simulink library "kif2"  (R2022a)
settings: Solver=VariableStepAuto  StartTime=0.0  StopTime=10.0  RelTol=1e-3
undefined symbols (not defined in the file or in its folder): DiscIntNeverNeededParam
libraries: $bdroot x9, spsThreePhaseDynamicLoadLib x1, spsThreePhaseSeriesRLCLoadLib x1, spsGroundLib x1, spsControlledCurrentSourceLib x1, spsFourierLib x1, spsPLLLib x1, spsSeriesRLCBranchLib x1, spsVoltageMeasurementLib x1, spsThreePhasePISectionLineLib x1, spsThreePhaseVIMeasurementLib x1
settings Model: Creator=Felhasználó  LastModifiedBy=Felhasználó

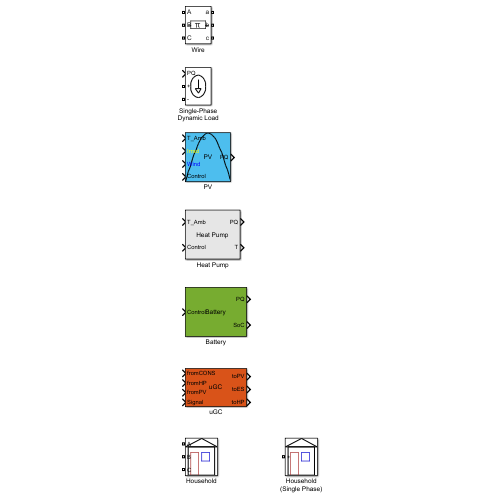
[thumbnail: Simulink's stored preview of the top-level diagram]
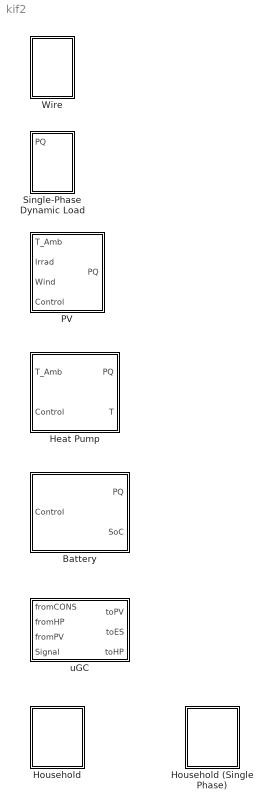
== system kif2 ==
  Battery : Subsystem  mask(Battery (Three Phase)){Cap=5000, SoCin=0.5, SoCmin=0.2, SoCmax=0.8, Pin=500, eta_in=0.95, Pout=-500, eta_out=0.95}
      mask prompts: Cap "Capacity (Wh)"; SoCin "Initial SoC (%)"; SoCmin "Min. SoC (%)"; SoCmax "Max. SoC (%)"; Pin "Max. charging power (W)"; eta_in "Charging efficiency (%)"; Pout "Max. discharging power (W)"; eta_out "Discharging efficiency (%)"
      mask help: This block models a battery.
      mask Display: disp('Battery');
  Heat Pump : Subsystem  mask(Heat Pump (Three Phase)){MFSystemSampleTime=0.05, tequiv=3, P_HP=3800, Tset=21, T_init=21, C=5940, H=192, ASHP=on, Mode=on, coeffs=[0.0012, -0.18, 8.6712], cosfi=0.9}
      mask prompts: MFSystemSampleTime "Simulink:blkprm_prompts:AllBlksSampleTime"; tequiv "Equivalent time (minutes)"; P_HP "Heat pump power (W)"; Tset "Set temperature (°C)"; T_init "Initial Temperature (°C)"; C "Building heat capacity (Wh/K)"; H "Building heat loss coefficient (W/K)"; ASHP "Air source heat pump"; Mode "Heating (/Cooling)"; coeffs "COP coefficients [a2 a1 a0]"; cosfi "Power factor (cosfi)"
      mask help: This block models an SG-Ready AHSP/WSHP/GSHP heat pump.
      mask TypeOptions MFSystemSampleTime: MATLAB Function/SystemSampleTime
      mask DialogControl MFSystemSampleTime Prompt: Sample time (-1 for inherited):
      mask Display: disp('Heat Pump');
  Household : Subsystem  mask(Household (Three Phase)){Ctag=CONSxx, Atag=Signal, Itag=Irradiation, Ttag=T_Amb, Wtag=Wind, HHtag=PQ_HHxx, HHtagv=local, PVtag=PQ_PVxx, PVtagv=local, EStag=PQ_ESxx, EStagv=local, HPtag=PQ_HPxx, HPtagv=local}
      mask prompts: Ctag "Consumption tag:"; Atag "Aggregator signal tag:"; Itag "Irradiation tag:"; Ttag "Temperature tag:"; Wtag "Wind tag:"; HHtag "Household:"; HHtagv "Simulink:blkprm_prompts:GotoTagVis"; PVtag "PV:"; PVtagv "Simulink:blkprm_prompts:GotoTagVis"; EStag "Battery:"; EStagv "Simulink:blkprm_prompts:GotoTagVis"; HPtag "Heat Pump:"; HPtagv "Simulink:blkprm_prompts:GotoTagVis"
      mask help: Represents a household, with PV, battery, heat pump and consumption.
      mask TypeOptions Ctag: Consumption/GotoTag
      mask TypeOptions Atag: Aggregator/GotoTag
      mask TypeOptions Itag: Irradiation/GotoTag
      mask TypeOptions Ttag: Temperature/GotoTag
      mask TypeOptions Wtag: Wind/GotoTag
      mask TypeOptions HHtag: PQ_HH/GotoTag
      mask TypeOptions HHtagv: PQ_HH/TagVisibility
      mask TypeOptions PVtag: PQ_PV/GotoTag
      mask TypeOptions PVtagv: PQ_PV/TagVisibility
      mask TypeOptions EStag: PQ_ES/GotoTag
      mask TypeOptions EStagv: PQ_ES/TagVisibility
      mask TypeOptions HPtag: PQ_HP/GotoTag
      mask TypeOptions HPtagv: PQ_HP/TagVisibility
      mask DialogControl InputTags Prompt: Inputs
      mask DialogControl WeatherTags Prompt: Weather
      mask DialogControl MeasurementTags Prompt: Measurement
      mask DialogControl HHtagv Prompt: Tag visibility:
      mask DialogControl PVtagv Prompt: Tag visibility:
      mask DialogControl EStagv Prompt: Tag visibility:
      mask DialogControl HPtagv Prompt: Tag visibility:
      mask Display:
      | plot([-5 -5 5 5 -5], [0 10 10 0 0]);
      | plot([-6 0 6 -6], [10 13 10 10]);
      | color('blue');
      | plot([0 3 3 0 0], [5 5 8 8 5]);
      | color('brown');
      | plot([-4 -1 -1 -4 -4], [0 0 8 8 0]);
  Household (Single Phase) : Subsystem  mask(Household (Single Phase)){Ctag=CONSxx, Atag=Signal, Itag=Irradiation, Ttag=T_Amb, Wtag=Wind, HHtag=PQ_HHxx, HHtagv=local, PVtag=PQ_PVxx, PVtagv=local, EStag=PQ_ESxx, EStagv=local, HPtag=PQ_HPxx, HPtagv=local}
      mask prompts: Ctag "Consumption tag:"; Atag "Aggregator signal tag:"; Itag "Irradiation tag:"; Ttag "Temperature tag:"; Wtag "Wind tag:"; HHtag "Household:"; HHtagv "Simulink:blkprm_prompts:GotoTagVis"; PVtag "PV:"; PVtagv "Simulink:blkprm_prompts:GotoTagVis"; EStag "Battery:"; EStagv "Simulink:blkprm_prompts:GotoTagVis"; HPtag "Heat Pump:"; HPtagv "Simulink:blkprm_prompts:GotoTagVis"
      mask help: Represents a Single Phase Household, with PV, battery, heat pump and consumption.
      mask TypeOptions Ctag: Consumption/GotoTag
      mask TypeOptions Atag: Aggregator/GotoTag
      mask TypeOptions Itag: Irradiation/GotoTag
      mask TypeOptions Ttag: Temperature/GotoTag
      mask TypeOptions Wtag: Wind/GotoTag
      mask TypeOptions HHtag: PQ_HH/GotoTag
      mask TypeOptions HHtagv: PQ_HH/TagVisibility
      mask TypeOptions PVtag: PQ_PV/GotoTag
      mask TypeOptions PVtagv: PQ_PV/TagVisibility
      mask TypeOptions EStag: PQ_ES/GotoTag
      mask TypeOptions EStagv: PQ_ES/TagVisibility
      mask TypeOptions HPtag: PQ_HP/GotoTag
      mask TypeOptions HPtagv: PQ_HP/TagVisibility
      mask DialogControl InputTags Prompt: Inputs
      mask DialogControl WeatherTags Prompt: Weather
      mask DialogControl MeasurementTags Prompt: Measurement
      mask DialogControl HHtagv Prompt: Tag visibility:
      mask DialogControl PVtagv Prompt: Tag visibility:
      mask DialogControl EStagv Prompt: Tag visibility:
      mask DialogControl HPtagv Prompt: Tag visibility:
      mask Display:
      | plot([-5 -5 5 5 -5], [0 10 10 0 0]);
      | plot([-6 0 6 -6], [10 13 10 10]);
      | color('blue');
      | plot([0 3 3 0 0], [5 5 8 8 5]);
      | color('brown');
      | plot([-4 -1 -1 -4 -4], [0 0 8 8 0]);
  PV : Subsystem  mask(PV (Three Phase)){P_STCm=2500, Ucoeff=[6.2 26.9], Kcoeff=[0.000005 0.00017 0.000149 -0.004702 -0.040465 -0.017237]}
      mask prompts: P_STCm "Peak Power (W)"; Ucoeff "Module temperature coefficients [u1 u0]"; Kcoeff "PV power dependence on irradiance and module temperature [k6 k5 k4 k3 k2 k1]"
      mask help: This block models a photovoltaic array.
      mask init:
      | U1 = Ucoeff(1);
      |     U0 = Ucoeff(2);
      |     k6 = Kcoeff(1);
      |     k5 = Kcoeff(2);
      |     k4 = Kcoeff(3);
      |     k3 = Kcoeff(4);
      |     k2 = Kcoeff(5);
      |     k1 = Kcoeff(6);
      mask Help: https://joint-research-centre.ec.europa.eu/photovoltaic-geographical-information-system-pvgis/getting-started-pvgis/pvgis-data-sources-calculation-methods_en
      mask Display:
      | disp('PV');
      | plot(-pi/2:0.1:pi/2, cos(-pi/2:0.1:pi/2));
  Single-Phase Dynamic Load : Subsystem  mask(Single-Phase Dynamic Load){Freq=50}
      mask prompts: Freq "Fundamental frequency (Hz):"
      mask help: This block models a PQ controlled single phase dynamic load.
      mask TypeOptions Freq: Fourier/Freq
      mask DialogControl ParameterGroupVar Prompt: PLL
      mask Display:
      | plot(-45,-45,45,45,[0,9,18,24,29,30,29,24,18,9,0,-9,-18,-24,-29,-30,-29,-24,-18,-9,0]*.9,[30,29,24,18,9,0,-9,-18,-24,-29,-30,-29,-24,-18,-9,0,9,18,24,29,30]*.9)
      | plot([0,0,10,0,-10,0]*1.1,[15,-5,-5,-15,-5,-5]*1.1)
  Wire : Subsystem  mask(Three-Phase Low Voltage Distribution Line){Length=0.03, Frequency=50, Resistances=[0.2968 0.4468], Inductances=[0.95359e-3  5.4671e-3], Capacitances=[12.458e-9 3.9055e-9], Vtag=V_Lxx, Vtagv=local, Itag=I_Lxx, Itagv=local}
      mask prompts: Length "Line length (km):"; Frequency "Frequency used for rlc specification (Hz):"; Resistances "Positive- and zero-sequence resistances (Ohms/km) [ r1  r0 ]:"; Inductances "Positive- and zero-sequence inductances (H/km) [ l1  l0 ]:"; Capacitances "Positive- and zero-sequence capacitances (F/km) [ c1 c0 ]:"; Vtag "V tag"; Vtagv "Visibility"; Itag "I tag"; Itagv "Visibility"
      mask help: This block models a low voltage distribution line with a Three-Phase PI Section Line, corresponding ports and V-I measurement.
      mask TypeOptions Length:
      | Three-Phase
      | PI Section Line/Length
      mask TypeOptions Frequency:
      | Three-Phase
      | PI Section Line/Frequency
      mask TypeOptions Resistances:
      | Three-Phase
      | PI Section Line/Resistances
      mask TypeOptions Inductances:
      | Three-Phase
      | PI Section Line/Inductances
      mask TypeOptions Capacitances:
      | Three-Phase
      | PI Section Line/Capacitances
      mask TypeOptions Vtag: Vmeas/GotoTag
      mask TypeOptions Vtagv: Vmeas/TagVisibility
      mask TypeOptions Itag: Imeas/GotoTag
      mask TypeOptions Itagv: Imeas/TagVisibility
      mask DialogControl Container3 Prompt: Measurements
      mask Display: block_icon('Three-Phase PI Section Line');
  uGC : Subsystem  mask(Microgrid Controller){}
      mask help: This block models a microgrid controller. It accepts aggregator signals, and controls PV, battery and heat pump.
      mask Display: disp('uGC');

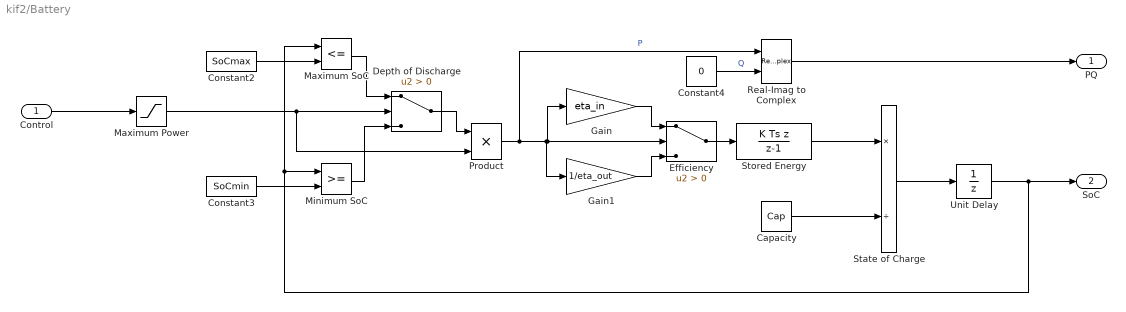
== system kif2/Battery ==
  Control : Inport
  Capacity : Constant  Value=Cap
  Constant2 : Constant  Value=SoCmax
  Constant3 : Constant  Value=SoCmin
  Constant4 : Constant  Value=0
  Depth of Discharge : Switch  Criteria=u2 > Threshold  SaturateOnIntegerOverflow=off  InputSameDT=off
  Efficiency : Switch  Criteria=u2 > Threshold  SaturateOnIntegerOverflow=off  InputSameDT=off
  Gain : Gain  Gain=eta_in
  Gain1 : Gain  Gain=1/eta_out
  Maximum Power : Saturate  UpperLimit=Pin  LowerLimit=Pout
  Maximum SoC : RelationalOperator  Operator=<=  OutDataTypeStr=boolean  RndMeth=Simplest  InputSameDT=off
  Minimum SoC : RelationalOperator  OutDataTypeStr=boolean  RndMeth=Simplest  InputSameDT=off
  Product : Product
  Real-Imag to Complex : RealImagToComplex
  State of Charge : Product  Inputs=*/
  Stored Energy : DiscreteIntegrator  IntegratorMethod=Integration: Backward Euler  InitialCondition=Cap*SoCin  SampleTime=1e-4  LimitOutput=on  UpperSaturationLimit=Cap  LowerSaturationLimit=0  ICPrevOutput=DiscIntNeverNeededParam  ICPrevScaledInput=DiscIntNeverNeededParam
  Unit Delay : UnitDelay  SampleTime=-1  HasFrameUpgradeWarning=on
  PQ : Outport
  SoC : Outport  Port=2
  wires:
  Control/1 -> Maximum Power/1
  Unit Delay/1 -> SoC/1, Maximum SoC/1, Minimum SoC/1
  Depth of Discharge/1 -> Product/1
  Product/1 -> Gain1/1, Gain/1, Efficiency/2, Real-Imag to Complex/1  "P"
  Constant4/1 -> Real-Imag to Complex/2  "Q"
  Maximum Power/1 -> Product/2, Depth of Discharge/2
  State of Charge/1 -> Unit Delay/1
  Constant2/1 -> Maximum SoC/2
  Stored Energy/1 -> State of Charge/1
  Maximum SoC/1 -> Depth of Discharge/1
  Capacity/1 -> State of Charge/2
  Minimum SoC/1 -> Depth of Discharge/3
  Constant3/1 -> Minimum SoC/2
  Real-Imag to Complex/1 -> PQ/1
  Efficiency/1 -> Stored Energy/1
  Gain/1 -> Efficiency/1
  Gain1/1 -> Efficiency/3

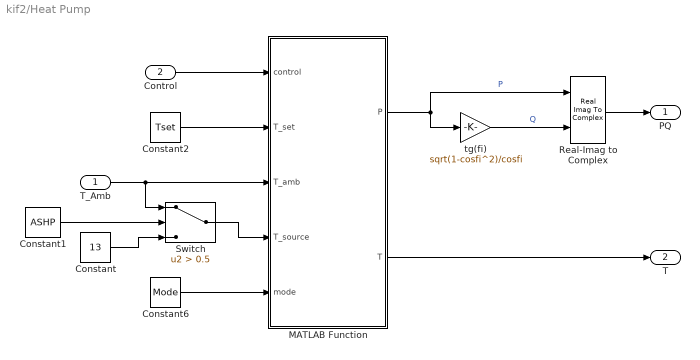
== system kif2/Heat Pump ==
  T_Amb : Inport
  Control : Inport  Port=2
  Constant : Constant  Value=13
  Constant1 : Constant  Value=ASHP
  Constant2 : Constant  Value=Tset
  Constant6 : Constant  Value=Mode
  MATLAB Function : MATLAB Function  TreatAsAtomicUnit=on  SystemSampleTime=MFSystemSampleTime
  Real-Imag to Complex : RealImagToComplex
  Switch : Switch  Criteria=u2 > Threshold  Threshold=0.5  SaturateOnIntegerOverflow=off  InputSameDT=off
  tg(fi) : Gain  Gain=sqrt(1-cosfi^2)/cosfi
  PQ : Outport
  T : Outport  Port=2
  wires:
  tg(fi)/1 -> Real-Imag to Complex/2  "Q"
  MATLAB Function/1(P) -> Real-Imag to Complex/1, tg(fi)/1  "P"
  T_Amb/1 -> Switch/1, MATLAB Function/3(T_amb)
  Constant2/1 -> MATLAB Function/2(T_set)
  Constant6/1 -> MATLAB Function/5(mode)
  Constant/1 -> Switch/3
  Switch/1 -> MATLAB Function/4(T_source)
  Constant1/1 -> Switch/2
  Control/1 -> MATLAB Function/1(control)
  MATLAB Function/2(T) -> T/1
  Real-Imag to Complex/1 -> PQ/1

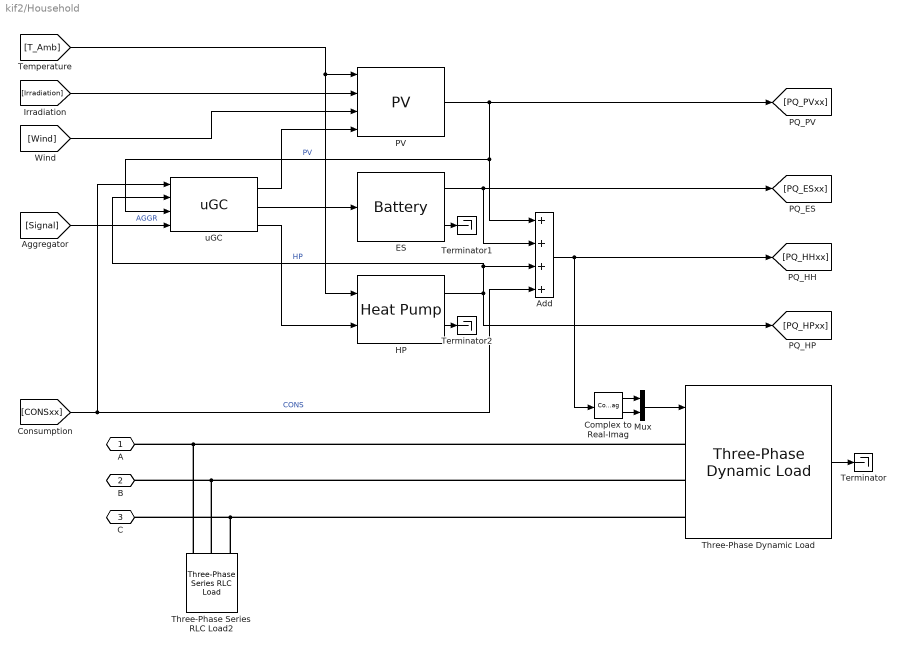
== system kif2/Household ==
  Add : Sum  Inputs=4
  Complex to Real-Imag : ComplexToRealImag
  ES : $bdroot/Battery  Cap=5000  SoCin=0.5  SoCmin=0.2  SoCmax=0.8  Pin=500  eta_in=0.95  Pout=-500  eta_out=0.95
  HP : $bdroot/Heat Pump  MFSystemSampleTime=0.05  tequiv=3  P_HP=3800  Tset=21  T_init=21  C=5940  H=192  ASHP=on  Mode=on  coeffs=[0.0012, -0.18, 8.6712]  cosfi=0.9
  Mux : Mux  Inputs=2
  PV : $bdroot/PV  P_STCm=2500  Ucoeff=[6.2 26.9]  Kcoeff=[0.000005 0.00017 0.000149 -0.004702 -0.040465 -0.017237]
  Terminator : Terminator
  Terminator1 : Terminator
  Terminator2 : Terminator
  Three-Phase Dynamic Load : spsThreePhaseDynamicLoadLib/Three-Phase Dynamic Load  NominalVoltage=[ 400 50 ]  ActiveReactivePowers=[0 0]  PositiveSequence=[0.994 -11.8]  ExternalControl=on  NpNq=[1.3 2]  TimeConstants="[0  0  0  0]"  MinimumVoltage=0.7  Tfilter=1e-4  LoadFlowParameters=[4,0,0,0,0]
      settings: SourceProductBaseCode=PS
  Three-Phase Series RLC Load2 : spsThreePhaseSeriesRLCLoadLib/Three-Phase Series RLC Load  LConnTagsString=A|B|C  Configuration=Y (grounded)  NominalVoltage=400  Vabc=[1e3 1e3 1e3]  Vabcp=[1e3 1e3 1e3]  NominalFrequency=50  UnbalancedPower=off  ActivePower=1  InductivePower=0  CapacitivePower=0  Pabc=[10e3 9e3 11e3]  QLabc=[100 90 110]  QCabc=[100 90 110]  Pabcp=[10e3 9e3 11e3]  QLabcp=[100 90 110]  QCabcp=[100 90 110]  Measurements=None  LoadType=constant Z
  uGC : $bdroot/uGC
  A : PMIOPort  Side=Left
  B : PMIOPort  Port=2  Side=Left
  C : PMIOPort  Port=3  Side=Left
  wires:
  Three-Phase Dynamic Load/1 -> Terminator/1
  Add/1 -> [PQ_HHxx], Complex to Real-Imag/1
  Complex to Real-Imag/1 -> Mux/1
  Complex to Real-Imag/2 -> Mux/2
  Mux/1 -> Three-Phase Dynamic Load/1
  PV/1 -> [PQ_PVxx], uGC/3, Add/1  "PV"
  [CONSxx] -> Add/4, uGC/1  "CONS"
  uGC/1 -> PV/4
  ES/1 -> [PQ_ESxx], Add/2
  HP/1 -> uGC/2, Add/3, [PQ_HPxx]  "HP"
  ES/2 -> Terminator1/1
  HP/2 -> Terminator2/1
  uGC/2 -> ES/1
  uGC/3 -> HP/2
  [Signal] -> uGC/4  "AGGR"
  [T_Amb] -> HP/1, PV/1
  [Irradiation] -> PV/2
  [Wind] -> PV/3
  connections:
  Three-Phase Dynamic Load/LConn1 -- A/RConn1 -- Three-Phase Series RLC Load2/LConn1
  Three-Phase Dynamic Load/LConn2 -- B/RConn1 -- Three-Phase Series RLC Load2/LConn2
  Three-Phase Dynamic Load/LConn3 -- C/RConn1 -- Three-Phase Series RLC Load2/LConn3

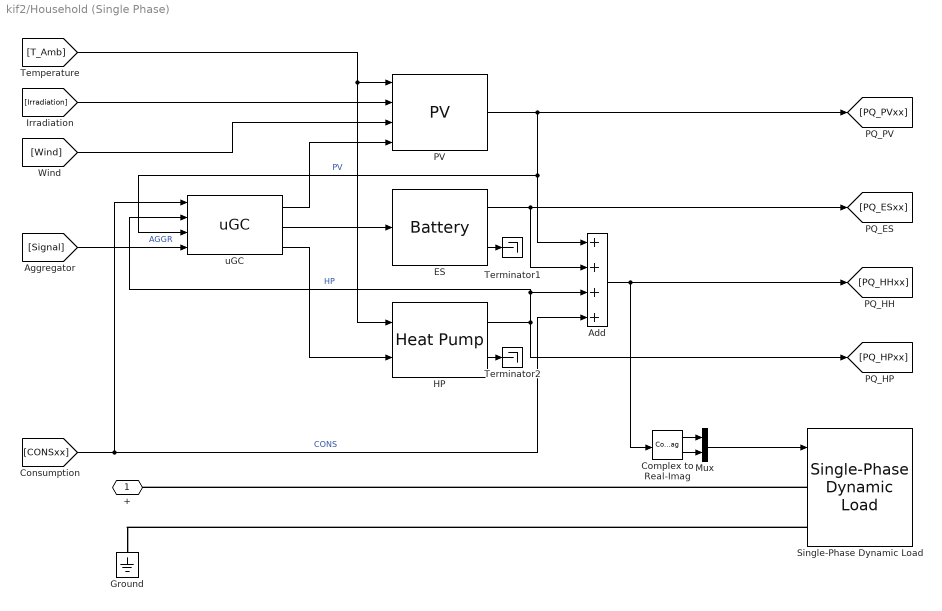
== system kif2/Household (Single Phase) ==
  Add : Sum  Inputs=4
  Complex to Real-Imag : ComplexToRealImag
  ES : $bdroot/Battery  Cap=5000  SoCin=0.5  SoCmin=0.2  SoCmax=0.8  Pin=500  eta_in=0.95  Pout=-500  eta_out=0.95
  Ground : spsGroundLib/Ground  LConnTagsString=a
  HP : $bdroot/Heat Pump  MFSystemSampleTime=0.05  tequiv=3  P_HP=3800  Tset=21  T_init=21  C=5940  H=192  ASHP=on  Mode=on  coeffs=[0.0012, -0.18, 8.6712]  cosfi=0.9
  Mux : Mux  Inputs=2
  PV : $bdroot/PV  P_STCm=2500  Ucoeff=[6.2 26.9]  Kcoeff=[0.000005 0.00017 0.000149 -0.004702 -0.040465 -0.017237]
  Single-Phase Dynamic Load : $bdroot/Single-Phase Dynamic Load  Freq=50
  Terminator1 : Terminator
  Terminator2 : Terminator
  uGC : $bdroot/uGC
  + : PMIOPort  Side=Left
  wires:
  [Wind] -> PV/3
  [Irradiation] -> PV/2
  [T_Amb] -> PV/1, HP/1
  [Signal] -> uGC/4  "AGGR"
  uGC/3 -> HP/2
  uGC/2 -> ES/1
  HP/2 -> Terminator2/1
  ES/2 -> Terminator1/1
  HP/1 -> [PQ_HPxx], Add/3, uGC/2  "HP"
  ES/1 -> Add/2, [PQ_ESxx]
  uGC/1 -> PV/4
  [CONSxx] -> Add/4, uGC/1  "CONS"
  PV/1 -> uGC/3, Add/1, [PQ_PVxx]  "PV"
  Mux/1 -> Single-Phase Dynamic Load/1
  Complex to Real-Imag/2 -> Mux/2
  Complex to Real-Imag/1 -> Mux/1
  Add/1 -> Complex to Real-Imag/1, [PQ_HHxx]
  connections:
  Single-Phase Dynamic Load/LConn1 -- +/RConn1
  Single-Phase Dynamic Load/LConn2 -- Ground/LConn1

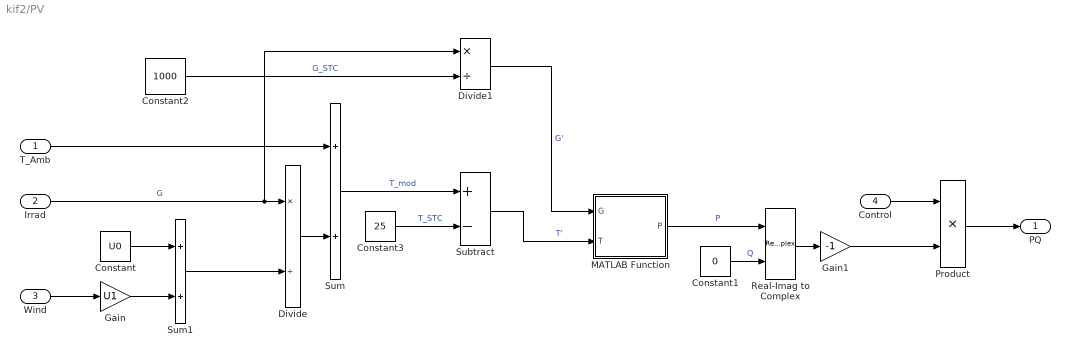
== system kif2/PV ==
  T_Amb : Inport
  Irrad : Inport  Port=2
  Wind : Inport  Port=3
  Control : Inport  Port=4
  Constant : Constant  Value=U0
  Constant1 : Constant  Value=0
  Constant2 : Constant  Value=1000
  Constant3 : Constant  Value=25
  Divide : Product  Inputs=*/
  Divide1 : Product  Inputs=*/
  Gain : Gain  Gain=U1
  Gain1 : Gain  Gain=-1
  MATLAB Function : MATLAB Function  TreatAsAtomicUnit=on
  Product : Product
  Real-Imag to Complex : RealImagToComplex
  Subtract : Sum  Inputs=+-
  Sum : Sum
  Sum1 : Sum
  PQ : Outport
  wires:
  Constant2/1 -> Divide1/2  "G_STC"
  Wind/1 -> Gain/1
  Irrad/1 -> Divide/1, Divide1/1  "G"
  T_Amb/1 -> Sum/1
  Constant3/1 -> Subtract/2  "T_STC"
  Sum/1 -> Subtract/1  "T_mod"
  Divide1/1 -> MATLAB Function/1(G)  "G'"
  Constant/1 -> Sum1/1
  Gain/1 -> Sum1/2
  Divide/1 -> Sum/2
  Sum1/1 -> Divide/2
  Subtract/1 -> MATLAB Function/2(T)  "T'"
  MATLAB Function/1(P) -> Real-Imag to Complex/1  "P"
  Constant1/1 -> Real-Imag to Complex/2  "Q"
  Control/1 -> Product/1
  Real-Imag to Complex/1 -> Gain1/1
  Product/1 -> PQ/1
  Gain1/1 -> Product/2

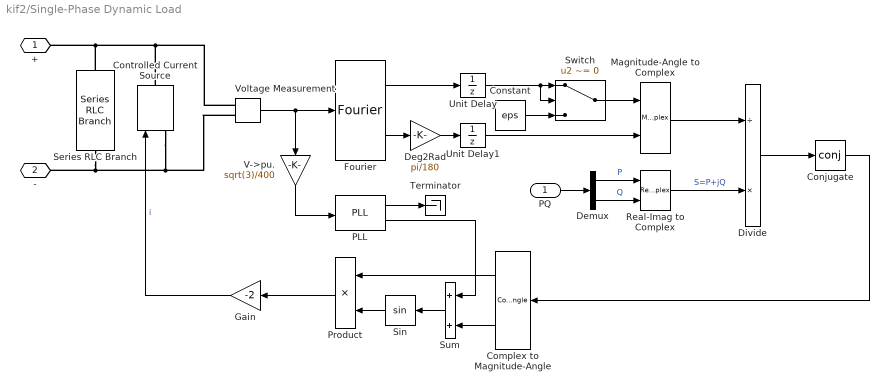
== system kif2/Single-Phase Dynamic Load ==
  PQ : Inport
  Complex to Magnitude-Angle : ComplexToMagnitudeAngle
  Conjugate : Math  Operator=conj  SignedPower=on  RndMeth=Zero
  Constant : Constant  Value=eps
  Controlled Current Source : spsControlledCurrentSourceLib/Controlled Current Source  Initialize=on  Source_Type=AC  Amplitude=0  Phase=0  Frequency=50  Measurements=None
  Deg2Rad : Gain  Gain=pi/180
  Demux : Demux  Outputs=2
  Divide : Product  Inputs=/*
  Fourier : spsFourierLib/Fourier  Freq=Freq  n=1  InInit=[400/sqrt(3), 0]  Ts=0
      settings: SourceProductBaseCode=PS
  Gain : Gain  Gain=-2
  Magnitude-Angle to Complex : MagnitudeAngleToComplex
  PLL : spsPLLLib/PLL  Fmin=45  Par_Init=[0, 50]  ParK=[180, 3200, 1]  TcD=1e-4  MaxRateChangeFreq=12  FilterCutOffFreq=25  Ts=0  AGC=on
      settings: SourceProductBaseCode=PS
  Product : Product
  Real-Imag to Complex : RealImagToComplex
  Series RLC Branch : spsSeriesRLCBranchLib/Series RLC Branch  LConnTagsString=__new0  RConnTagsString=__new0  BranchType=R  Resistance=1e6  Inductance=1e-3  SetiL0=off  InitialCurrent=0  Capacitance=1e-6  Setx0=off  InitialVoltage=0  Measurements=None
  Sin : Trigonometry
  Sum : Sum
  Switch : Switch  Criteria=u2 ~= 0  SaturateOnIntegerOverflow=off  InputSameDT=off
  Terminator : Terminator
  Unit Delay : UnitDelay  SampleTime=-1  HasFrameUpgradeWarning=on
  Unit Delay1 : UnitDelay  SampleTime=-1  HasFrameUpgradeWarning=on
  V->pu. : Gain  Gain=sqrt(3)/400
  Voltage Measurement : spsVoltageMeasurementLib/Voltage Measurement  PhasorSimulation=off  OutputType=Complex  PSBequivalent=0
  + : PMIOPort  Side=Left
  - : PMIOPort  Port=2  Side=Left
  wires:
  Divide/1 -> Conjugate/1
  Fourier/1 -> Unit Delay/1
  Complex to Magnitude-Angle/1 -> Product/1
  Magnitude-Angle to Complex/1 -> Divide/1
  Sum/1 -> Sin/1
  PQ/1 -> Demux/1
  Unit Delay1/1 -> Magnitude-Angle to Complex/2
  Voltage Measurement/1 -> V->pu./1, Fourier/1
  Constant/1 -> Switch/3
  PLL/1 -> Terminator/1
  Demux/1 -> Real-Imag to Complex/1  "P"
  Unit Delay/1 -> Switch/2, Switch/1
  Complex to Magnitude-Angle/2 -> Sum/2
  Sin/1 -> Product/2
  Product/1 -> Gain/1
  Real-Imag to Complex/1 -> Divide/2  "S=P+jQ"
  Fourier/2 -> Deg2Rad/1
  Conjugate/1 -> Complex to Magnitude-Angle/1
  Gain/1 -> Controlled Current Source/1  "i"
  Switch/1 -> Magnitude-Angle to Complex/1
  Demux/2 -> Real-Imag to Complex/2  "Q"
  PLL/2 -> Sum/1
  Deg2Rad/1 -> Unit Delay1/1
  V->pu./1 -> PLL/1
  connections:
  Voltage Measurement/LConn2 -- Controlled Current Source/LConn1 -- -/RConn1 -- Series RLC Branch/RConn1
  Voltage Measurement/LConn1 -- +/RConn1 -- Series RLC Branch/LConn1 -- Controlled Current Source/RConn1

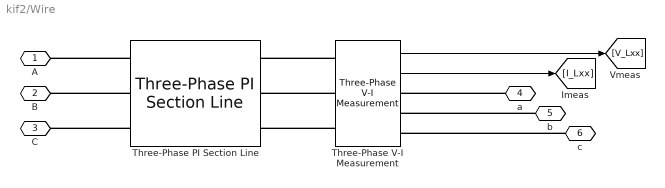
== system kif2/Wire ==
  Three-Phase PI Section Line : spsThreePhasePISectionLineLib/Three-Phase PI Section Line  LConnTagsString=a|b|c  RConnTagsString=A|B|C  Length=Length  Frequency=Frequency  Resistances=Resistances  Inductances=Inductances  Capacitances=Capacitances
  Three-Phase V-I Measurement : spsThreePhaseVIMeasurementLib/Three-Phase V-I Measurement  VoltageMeasurement=phase-to-ground  SetLabelV=off  LabelV=Vabc  Vpu=off  VpuLL=off  CurrentMeasurement=yes  SetLabelI=off  LabelI=Iabc  Ipu=off  Pbase=100e6  Vbase=500e3  OutputType=Complex  PhasorSimulation=off  PSBequivalent=0
  A : PMIOPort  Side=Left
  B : PMIOPort  Port=2  Side=Left
  C : PMIOPort  Port=3  Side=Left
  a : PMIOPort  Port=4  Side=Right
  b : PMIOPort  Port=5  Side=Right
  c : PMIOPort  Port=6  Side=Right
  wires:
  Three-Phase V-I Measurement/1 -> [V_Lxx]
  Three-Phase V-I Measurement/2 -> [I_Lxx]
  connections:
  c/RConn1 -- Three-Phase V-I Measurement/RConn3
  Three-Phase PI Section Line/LConn3 -- C/RConn1
  Three-Phase V-I Measurement/LConn3 -- Three-Phase PI Section Line/RConn3
  b/RConn1 -- Three-Phase V-I Measurement/RConn2
  Three-Phase V-I Measurement/LConn2 -- Three-Phase PI Section Line/RConn2
  a/RConn1 -- Three-Phase V-I Measurement/RConn1
  Three-Phase PI Section Line/LConn2 -- B/RConn1
  Three-Phase PI Section Line/LConn1 -- A/RConn1
  Three-Phase V-I Measurement/LConn1 -- Three-Phase PI Section Line/RConn1

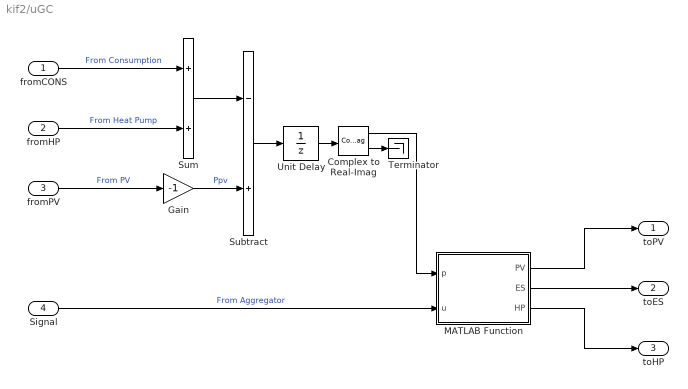
== system kif2/uGC ==
  fromCONS : Inport
  fromHP : Inport  Port=2
  fromPV : Inport  Port=3
  Signal : Inport  Port=4
  Complex to Real-Imag : ComplexToRealImag
  Gain : Gain  Gain=-1
  MATLAB Function : MATLAB Function  TreatAsAtomicUnit=on
  Subtract : Sum  Inputs=-+
  Sum : Sum
  Terminator : Terminator
  Unit Delay : UnitDelay  SampleTime=-1  HasFrameUpgradeWarning=on
  toPV : Outport
  toES : Outport  Port=2
  toHP : Outport  Port=3
  wires:
  Sum/1 -> Subtract/1
  Subtract/1 -> Unit Delay/1
  MATLAB Function/3(HP) -> toHP/1
  MATLAB Function/1(PV) -> toPV/1
  MATLAB Function/2(ES) -> toES/1
  fromCONS/1 -> Sum/1  "From Consumption"
  fromHP/1 -> Sum/2  "From Heat Pump"
  fromPV/1 -> Gain/1  "From PV"
  Signal/1 -> MATLAB Function/2(u)  "From Aggregator"
  Gain/1 -> Subtract/2  "Ppv"
  Unit Delay/1 -> Complex to Real-Imag/1
  Complex to Real-Imag/1 -> MATLAB Function/1(p)
  Complex to Real-Imag/2 -> Terminator/1

== matlab function kif2/PV/MATLAB Function ==
  data: G input; P output; T input; P_STCm parameter; k1 parameter; k2 parameter; k3 parameter; k4 parameter; k5 parameter; k6 parameter
function P = fcn(G,T, P_STCm, k1, k2, k3, k4, k5, k6)
    if G < eps
        P = 0;
    else
        P = G*(P_STCm + k1*log(G) + k2*log(G)^2 + k3*T + k4*T*log(G) + k5*T*log(G)^2 + k6*T^2);
    end
end

== matlab function kif2/Heat Pump/MATLAB Function ==
  data: P output; control input; T_set input; T_amb input; T_source input; mode input; T output; P_HP parameter; H parameter; C parameter; coeffs parameter; T_init parameter; tequiv parameter
% OFF = 1
% NORMAL = 2
% ON = 3
% SUPERHEAT_A = 4
% SUPERHEAT_B = 5

function [P, T] = fcn(control, T_set, T_amb, T_source, mode, P_HP, H, C, coeffs, T_init, tequiv)
    HYST = 0.5;
    HYST_adj = 1;
    min_run_time = 3;
    min_pause_time = 6;
    T_sink = 45;
    
    persistent pause_time;
    if isempty(pause_time)
        pause_time = 0;
    end
    persistent run_time;
    if isempty(run_time)
        run_time = 0;
    end
    persistent on;
    if isempty(on)
        on = false;
    end
    persistent prev_control;
    if isempty(prev_control)
        prev_control = 2;
    end
    
    persistent T_in;
    if isempty(T_in)
        T_in = T_init;
    end
    
    %initial values
    Q_HP = 0;
    %default hysteresis
    T_min = T_set - HYST;
    T_max = T_set + HYST;
    
    if (mode) %heating
        %adjust histeresis based on control
        if (control == 3 || control >= 4)
            T_min = T_set;
            T_max = T_set + HYST + HYST_adj;
        end
        %switch on/off
        if (~on && ...
                pause_time >= min_pause_time && ...
                control ~= 1 && ...
                (T_in < T_min || (control >= 4 && prev_control < 4)))
            on = true;
            run_time = 0;
        elseif (on && ...
                run_time >= min_run_time && ...
                (T_in > T_max || control == 1))
            on = false;
            pause_time = 0;
        end
        %determine P and Q
        if (on)
            COP = polyval(coeffs, T_sink - T_source);
            Q_HP = P_HP * COP;
            P = P_HP;
            run_time = run_time + tequiv;
        else
            P = 0;
            pause_time = pause_time + tequiv;
        end
    else %cooling
        %adjust histeresis based on control
        if (control == 3 || control >= 4)
            T_min = T_set - HYST - HYST_adj;
            T_max = T_set;
        end
        %switch on/off
        if (~on && ...
                pause_time >= min_pause_time && ...
                control ~= 1 && ...
                (T_in > T_max || (control >= 4 && prev_control < 4)))
            on = true;
            run_time = 0;
        elseif (on && ...
                run_time >= min_run_time && ...
                (T_in < T_min || control == 1))
            on = false;
            pause_time = 0;
        end
        %determine P and Q
        if (on)
            COP = polyval(coeffs, T_source - T_sink) - 1;
            Q_HP = - P_HP * COP;
            P = P_HP;
            run_time = run_time + tequiv;
        else
            P = 0;
            pause_time = pause_time + tequiv;
        end
    end
    %simulate diff. eq.
    h = tequiv/60;
    T_in = T_in + h * (-H/C*(T_in - T_amb) + Q_HP/C);
    prev_control = control;
    T = T_in;
end

== matlab function kif2/uGC/MATLAB Function ==
  data: p input; u input; PV output; ES output; HP output
function [PV, ES, HP] = fcn(p, u)
    switch u
        case -1 % down
            PV = 1;
            ES = -inf;
            HP = 1;
        case 0 % normal
            PV = 1;
            ES = p;
            HP = 2;
        case 1 % up
            PV = 0;
            ES = inf;
            HP = 4;
        otherwise % normal
            PV = 1;
            ES = p;
            HP = 2;
    end
end
